simulink model "AFG_s1v1"  (R2022b)
settings: Solver=ode45  StartTime=0.0  StopTime=inf  RelTol=1e-3  EnableMultiTasking=on
values from neighbouring files (symbols this model uses):
  axle_rate_limit = 1    [call_AFG4hil_s1v1.m]
  BRAKE = [1 1 1 1 1 1 1 1]/8'    [call_AFG4hil_s1v1.m]    (also in call_AFG_s1v1.m)
  brake_lag = 0.002    [call_AFG_s1v1.m]
  brake_rate = 5000    [call_AFG_s1v1.m]
  DRIVE = [0.25 0.25  0 0 0 0 0.25 0.25]/1'    [call_AFG4hil_s1v1.m]    (also in call_AFG_s1v1.m)
  Kad = 0.0    (= 0)    [call_AFG4hil_s1v1.m]
  Kai = 0.05    [call_AFG4hil_s1v1.m]
  Kap = 0.1    [call_AFG4hil_s1v1.m]
  KDspd = 0.1    [call_AFG4hil_s1v1.m]    (also in call_AFG_s1v1.m = 0)
  KIspd = 0.1    [call_AFG4hil_s1v1.m]    (also in call_AFG_s1v1.m = 0)
  KPspd = 10    [call_AFG4hil_s1v1.m]    (also in call_AFG_s1v1.m = 20)
  Lspd = -7    [call_AFG4hil_s1v1.m]
  Nspd = 10    [call_AFG4hil_s1v1.m]
  RW = 0.499    [call_AFG4hil_s1v1.m]    (also in call_AFG_s1v1.m)
  Tb = 0.002    [call_AFG_s1v1.m]
  TRACK = temptrack    [article.m]    (also in calculate_offtrack.m; call_AFG4hil_s1v1.m = trackgen4(2,50); call_AFG_s1v1.m = trackgen4(2,50); tracktest.m)
  Tst = 0.05    [call_AFG4hil_s1v1.m]    (also in call_AFG_s1v1.m = 0.02)
  Uspd = 5    [call_AFG4hil_s1v1.m]
  vconst = 15*kph    (= 4.16666666667)    [call_AFG4hil_s1v1.m]    (also in call_AFG_s1v1.m = 5.55555555556)
undefined symbols (not defined in the file or in its folder): PARSa, PARSu, TOTALMASS
libraries: CarMaker4SL x154, slpidlib x2, TruckMaker4SL x1, simulink x1
(part 1 of 3)
settings Model: Creator=fh  LastModifiedBy=14668
settings SolverCC: AlgebraicLoopSolver=TrustRegion
settings DataIOCC: LimitDataPoints=on  SaveFormat=Array  ReturnWorkspaceOutputs=off  SignalLoggingName=sigsOut
settings OptimizationCC: BooleanDataType=off  ExpressionDepthLimit=2147483647  InitFltsAndDblsToZero=on  LifeSpan=inf
settings DebuggingCC: SaveWithParameterizedLinksMsg=none  UnderspecifiedInitializationDetection=Classic  MergeDetectMultiDrivingBlocksExec=none  SignalResolutionControl=TryResolveAllWithWarning  MultiTaskDSMMsg=warning  MultiTaskCondExecSysMsg=none  FcnCallInpInsideContextMsg=warning  UnconnectedInputMsg=warning  UnconnectedOutputMsg=warning  UnconnectedLineMsg=warning  StateNameClashWarn=warning  SFUnexpectedBacktrackingDiag=warning  SFNoUnconditionalDefaultTransitionDiag=warning  SFMachineParentedDataDiag=warning  ArithmeticOperatorsInVariantConditions=warning
settings HardwareCC: ProdBitPerPointer=32  ProdBitPerSizeT=32  ProdBitPerPtrDiffT=32  ProdLargestAtomicFloat=None  ProdIntDivRoundTo=Undefined  ProdEndianess=Unspecified  ProdWordSize=32  ProdHWDeviceType=32-bit Generic  TargetUnknown=on
settings ModelReferenceCC: EnableRefExpFcnMdlSchedulingChecks=on  PropagateSignalLabelsOutOfModel=off
settings SFSimCC: SimUseLocalCustomCode=off  CustomCodeUndefinedFunction=UseInterfaceOnly
settings RTWCC: RTWUseLocalCustomCode=off
settings CodeAppCC: MaxIdLength=63  StateflowObjectComments=on
settings GRTTargetCC: TargetFcnLib=ansi_tfl_tmw.mat  TargetLangStandard=C89/C90 (ANSI)  CombineOutputUpdateFcns=off  GRTInterface=on
settings ConfigComp: CovMetricSettings=dw  CovSaveCumulativeToWorkspaceVar=on  CovSaveSingleToWorkspaceVar=on  CovExternalEMLEnable=off

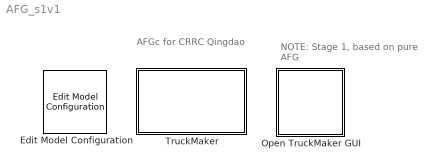
== system AFG_s1v1 ==
  note: AFGc for CRRC Qingdao
  note: NOTE:
      | Stage 1, based on pure AFG
  Edit Model Configuration : TruckMaker4SL/Edit Model Configuration  SFunctionModules=''
  Open TruckMaker GUI : Subsystem  LoadFcn=if ~length(which('cmself')), cmenv; end
      settings: OpenFcn=cmblockmagic('gui_fix_display'); TM_Simulink
      mask Display: image(imread('TruckMakerGUI.png'));
  TruckMaker : Subsystem  TreatAsAtomicUnit=on
      mask Display: image(imread('TruckMakerSys.png'));

== system AFG_s1v1/Open TruckMaker GUI ==
  S-Function : S-Function  FunctionName=cm_gui  SFunctionDeploymentMode=off  EnableBusSupport=off

== system AFG_s1v1/TruckMaker ==
  note: main code in IPG Vehicle
  CM_FIRST : Subsystem
  CM_LAST : Subsystem
  DrivMan : Subsystem
  Ground : Ground
  IPG Vehicle : Subsystem  TreatAsAtomicUnit=on
  Terminator : Terminator
  VehicleControl : Subsystem
  wires:
  VehicleControl/2(Vhcl.Model.Source) -> IPG Vehicle/2(Vhcl.Model.Source)
  VehicleControl/7(VhclCtrl.PT) -> IPG Vehicle/7(VhclCtrl.PT)
  VehicleControl/6(VhclCtrl.Brake) -> IPG Vehicle/6(VhclCtrl.Brake)
  VehicleControl/5(Vhcl.Misc) -> IPG Vehicle/5(Vhcl.Misc)
  VehicleControl/4(Vhcl.Wheel.In) -> IPG Vehicle/4(Vhcl.Wheel.In)
  VehicleControl/3(VhclCtrl.Steering) -> IPG Vehicle/3(VhclCtrl.Steering)
  VehicleControl/1(Sync_Out) -> IPG Vehicle/1(Sync_In)
  IPG Vehicle/1(Sync_Out) -> CM_LAST/1(Sync_In)
  Ground/1 -> CM_FIRST/1(Sync_In)
  CM_LAST/1(Sync_Out) -> Terminator/1
  CM_FIRST/1(Sync_Out) -> DrivMan/1(Sync_In)
  CM_FIRST/2(Env.Misc) -> DrivMan/2(Env.Misc)
  DrivMan/1(Sync_Out) -> VehicleControl/1(Sync_In)
  DrivMan/2(DrivMan.Out) -> VehicleControl/2(DrivMan.In)

== system AFG_s1v1/TruckMaker/CM_FIRST ==
  Sync_In : Inport
  BusCreator1 : BusCreator  Inputs=8
  BusCreator2 : BusCreator  Inputs=6
  Demux1 : Demux  Outputs=14
      settings: DisplayOption=none
  Environment : S-Function  FunctionName=TM_Sfun  Parameters='Environment'  SFunctionDeploymentMode=off  EnableBusSupport=off
  IoIn : S-Function  FunctionName=TM_Sfun  Parameters='IoIn'  SFunctionDeploymentMode=off  EnableBusSupport=off
  Terminator : Terminator
  Sync_Out : Outport
  Env.Misc : Outport  Port=2
  wires:
  BusCreator2/1 -> Terminator/1  "IF Environment (in)"
  BusCreator1/1 -> Env.Misc/1
  Demux1/14 -> BusCreator2/6  "Env sRoad"
  Demux1/13 -> BusCreator2/5  "Env PoI_GCS Elev"
  Demux1/12 -> BusCreator2/4  "Env PoI_GCS Lat"
  Demux1/11 -> BusCreator2/3  "Env PoI_GCS Long"
  Demux1/10 -> BusCreator2/2  "Env Time"
  Demux1/9 -> BusCreator2/1  "Env yDay"
  Demux1/8 -> BusCreator1/8  "Env WindVel_tot z"
  Demux1/7 -> BusCreator1/7  "Env WindVel_tot y"
  Demux1/6 -> BusCreator1/6  "Env WindVel_tot x"
  Demux1/5 -> BusCreator1/5  "Env SolarRadiation"
  Demux1/4 -> BusCreator1/4  "Env AirHumidity"
  Demux1/3 -> BusCreator1/3  "Env AirPressure"
  Demux1/2 -> BusCreator1/2  "Env AirDensity"
  Demux1/1 -> BusCreator1/1  "Env Temperature"
  Environment/2 -> Demux1/1
  Environment/1 -> Sync_Out/1
  IoIn/1 -> Environment/1
  Sync_In/1 -> IoIn/1

== system AFG_s1v1/TruckMaker/CM_LAST ==
  Sync_In : Inport
  CM_User : S-Function  FunctionName=TM_Sfun  Parameters='CM_User'  SFunctionDeploymentMode=off  EnableBusSupport=off
  IoOut : S-Function  FunctionName=TM_Sfun  Parameters='IoOut'  SFunctionDeploymentMode=off  EnableBusSupport=off
  Sync_Out : Outport
  wires:
  IoOut/1 -> Sync_Out/1
  CM_User/1 -> IoOut/1
  Sync_In/1 -> CM_User/1

== system AFG_s1v1/TruckMaker/DrivMan ==
  note: There's rarely a reason to override DrivMan signals.
      | Use the VehicleControl interface for this purpose.
  Sync_In : Inport
  Env.Misc : Inport  Port=2
  BusCreator : BusCreator  Inputs=17
  Demux : Demux  Outputs=17
      settings: DisplayOption=none
  DrivMan : S-Function  FunctionName=TM_Sfun  Parameters='DrivMan'  SFunctionDeploymentMode=off  EnableBusSupport=off
  Sync_Out : Outport
  DrivMan.Out : Outport  Port=2
  wires:
  Demux/17 -> BusCreator/17  "DrivMan Steering Trq"
  Demux/16 -> BusCreator/16  "DrivMan Steering AngAcc"
  Demux/15 -> BusCreator/15  "DrivMan Steering AngVel"
  Demux/14 -> BusCreator/14  "DrivMan Steering Ang"
  Demux/13 -> BusCreator/13  "DrivMan Gas"
  Demux/12 -> BusCreator/12  "DrivMan Clutch"
  Demux/11 -> BusCreator/11  "DrivMan BrakePark"
  Demux/10 -> BusCreator/10  "DrivMan Brake"
  Demux/9 -> BusCreator/9  "DrivMan GearNo"
  Demux/8 -> BusCreator/8  "DrivMan SelectorCtrl"
  Demux/7 -> BusCreator/7  "DrivMan UserSignal4"
  Demux/6 -> BusCreator/6  "DrivMan UserSignal3"
  Demux/5 -> BusCreator/5  "DrivMan UserSignal2"
  Demux/4 -> BusCreator/4  "DrivMan UserSignal1"
  Demux/3 -> BusCreator/3  "DrivMan UserSignal0"
  Demux/2 -> BusCreator/2  "DrivMan Key"
  Demux/1 -> BusCreator/1  "DrivMan SST"
  Env.Misc/1 -> DrivMan/2
  Sync_In/1 -> DrivMan/1
  DrivMan/1 -> Sync_Out/1
  BusCreator/1 -> DrivMan.Out/1
  DrivMan/2 -> Demux/1

== system AFG_s1v1/TruckMaker/IPG Vehicle ==
  Sync_In : Inport
  Vhcl.Model.Source : Inport  Port=2
  VhclCtrl.Steering : Inport  Port=3
  Vhcl.Wheel.In : Inport  Port=4
  Vhcl.Misc : Inport  Port=5
  VhclCtrl.Brake : Inport  Port=6
  VhclCtrl.PT : Inport  Port=7
  AFGc : Subsystem
  Brake : Subsystem
  CarAndTrailer : Subsystem
  DAQ for addtional VIS and DEBUG : Subsystem
  PowerTrain : Subsystem
  Stop Simulation : Stop
  VehicleSource_BuiltIn : simulink/Logic and Bit Operations/Compare To Constant  relop=~=  const=1  OutDataTypeStr=boolean  ZeroCross=off
  Sync_Out : Outport
  wires:
  VhclCtrl.PT/1 -> PowerTrain/3(VhclCtrl.PT)
  Brake/1(Sync_Out) -> PowerTrain/1(Sync_In)
  CarAndTrailer/1(Sync_Out) -> Brake/1(Sync_In)
  CarAndTrailer/2(Brake.IF.In) -> Brake/2(Brake.IF.In)
  VhclCtrl.Brake/1 -> Brake/3(VhclCtrl.Brake)
  PowerTrain/1(Sync_Out) -> Sync_Out/1
  Vhcl.Misc/1 -> CarAndTrailer/4(Vhcl.Misc)
  Vhcl.Wheel.In/1 -> CarAndTrailer/3(Vhcl.Wheel.In)
  VhclCtrl.Steering/1 -> CarAndTrailer/2(VhclCtrl.Steering)
  Sync_In/1 -> CarAndTrailer/1(Sync_In)
  Vhcl.Model.Source/1 -> VehicleSource_BuiltIn/1
  VehicleSource_BuiltIn/1 -> Stop Simulation/1
  Brake/2(Vhcl.Wheel.PT) -> PowerTrain/2(Vhcl.Wheel.PT)
  AFGc/1(tractor brake1) -> Brake/4(tractor brake)

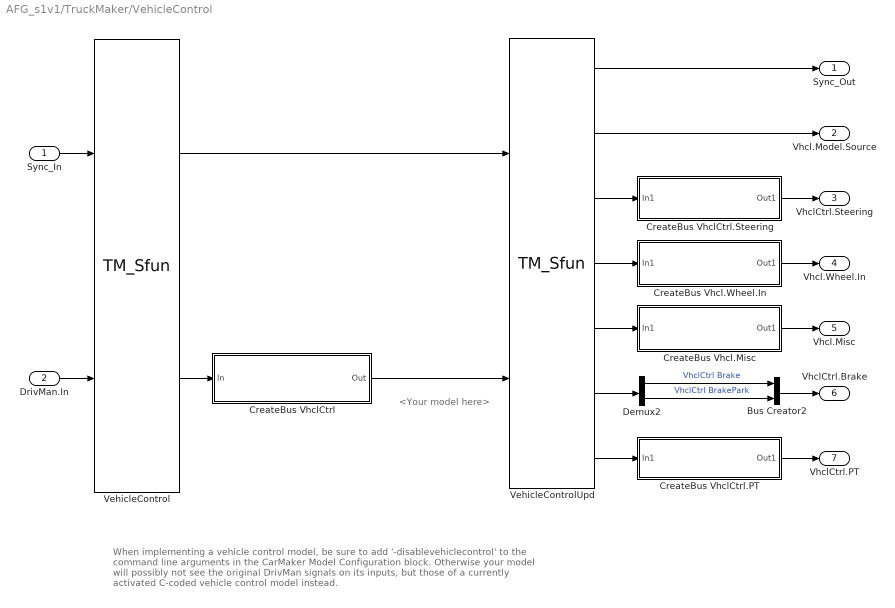
== system AFG_s1v1/TruckMaker/VehicleControl ==
  note: <Your model here>
  note: When implementing a vehicle control model,
      | be sure to add '-disablevehiclecontrol' to the command line arguments
      | in the CarMaker Model Configuration block.
      | Otherwise your model will possibly not see the original DrivMan signals
      | on its inputs, but those of a currently activated C-coded vehicle control model instead.
  Sync_In : Inport
  DrivMan.In : Inport  Port=2
  Bus Creator2 : BusCreator  Inputs=2
  CreateBus Vhcl.Misc : Subsystem
  CreateBus Vhcl.Wheel.In : Subsystem
  CreateBus VhclCtrl : Subsystem
  CreateBus VhclCtrl.PT : Subsystem
  CreateBus VhclCtrl.Steering : Subsystem
  Demux2 : Demux  Outputs=2
      settings: DisplayOption=none
  VehicleControl : S-Function  FunctionName=TM_Sfun  Parameters='VehicleControl'  SFunctionDeploymentMode=off  EnableBusSupport=off
  VehicleControlUpd : S-Function  FunctionName=TM_Sfun  Parameters='VehicleControlUpd'  SFunctionDeploymentMode=off  EnableBusSupport=off
  Sync_Out : Outport
  Vhcl.Model.Source : Outport  Port=2
  VhclCtrl.Steering : Outport  Port=3
  Vhcl.Wheel.In : Outport  Port=4
  Vhcl.Misc : Outport  Port=5
  VhclCtrl.Brake : Outport  Port=6
  VhclCtrl.PT : Outport  Port=7
  wires:
  VehicleControlUpd/2 -> Vhcl.Model.Source/1
  VehicleControlUpd/4 -> CreateBus Vhcl.Wheel.In/1(In1)
  VehicleControlUpd/5 -> CreateBus Vhcl.Misc/1(In1)
  VehicleControlUpd/6 -> Demux2/1
  VehicleControlUpd/7 -> CreateBus VhclCtrl.PT/1(In1)
  VehicleControlUpd/3 -> CreateBus VhclCtrl.Steering/1(In1)
  CreateBus Vhcl.Misc/1(Out1) -> Vhcl.Misc/1
  CreateBus Vhcl.Wheel.In/1(Out1) -> Vhcl.Wheel.In/1
  DrivMan.In/1 -> VehicleControl/2
  CreateBus VhclCtrl/1(Out) -> VehicleControlUpd/2
  VehicleControl/1 -> VehicleControlUpd/1
  VehicleControl/2 -> CreateBus VhclCtrl/1(In)
  Sync_In/1 -> VehicleControl/1
  CreateBus VhclCtrl.PT/1(Out1) -> VhclCtrl.PT/1
  Bus Creator2/1 -> VhclCtrl.Brake/1
  CreateBus VhclCtrl.Steering/1(Out1) -> VhclCtrl.Steering/1
  VehicleControlUpd/1 -> Sync_Out/1
  Demux2/2 -> Bus Creator2/2  "VhclCtrl BrakePark"
  Demux2/1 -> Bus Creator2/1  "VhclCtrl Brake"

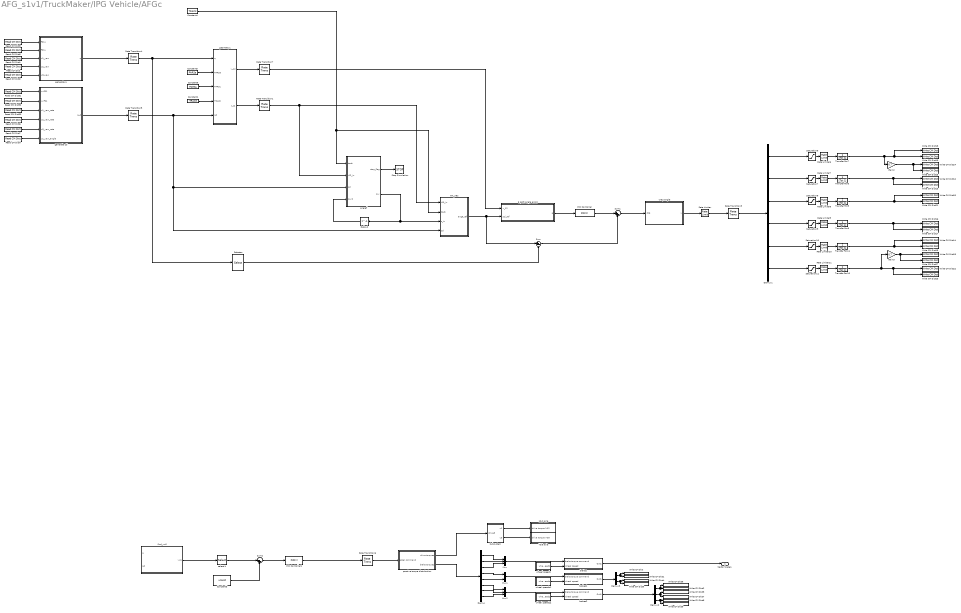
== system AFG_s1v1/TruckMaker/IPG Vehicle/AFGc ==
  1&2 axle : Subsystem
  6 path angle errors : MATLAB Function  TreatAsAtomicUnit=on
  7&8 axle : Subsystem
  Constant1 : Constant  Value=TRACK
  Constant3 : Constant  Value=vconst
  Constant4 : Constant  Value=TRACK
  Constant5 : Constant  Value=PARSa
  Constant6 : Constant  Value=PARSu
  Delay2 : Delay  DelayLength=1
  Demux : Demux  Outputs=8
  Demux1 : Demux  Outputs=6
  Demux2 : Demux  Outputs=3
  Demux3 : Demux  Outputs=2
  Gain2 : Gain  Gain=0.7
  Gain3 : Gain  Gain=0.7
  Mux : Mux  Inputs=3
  Mux1 : Mux  Inputs=2
  Mux2 : Mux  Inputs=3
  PID Controller : slpidlib/PID Controller  Controller=PID  Form=Parallel  TimeDomain=Discrete-time  UseExternalTs=off  SampleTime=-1  IntegratorMethod=Forward Euler  FilterMethod=Forward Euler  ControllerParametersSource=internal  P=Kap  I=Kai  UseKiTs=off  D=Kad  N=100  UseFilter=off  TunerSelectOption=Transfer Function Based (PID Tuner App)  InitialConditionSource=internal  InitialConditionForIntegrator=0  InitialConditionForFilter=0  DifferentiatorICPrevScaledInput=0  ExternalReset=none  TrackingMode=off  Kt=1  LimitOutput=on  SatLimitsSource=internal  UpperSaturationLimit=0.1  LowerSaturationLimit=-0.1  LinearizeAsGain=on  AntiWindupMode=clamping  Kb=1  LimitIntegrator=off  UpperIntegratorSaturationLimit=inf  LowerIntegratorSaturationLimit=-inf  POutMin=[]  POutMax=[]  IOutMin=[]  IOutMax=[]  DOutMin=[]  DOutMax=[]  NOutMin=[]  NOutMax=[]  SumOutMin=[]  SumOutMax=[]  SaturationOutMin=[]  SaturationOutMax=[]  PParamMin=[]  PParamMax=[]  IParamMin=[]  IParamMax=[]  DParamMin=[]  DParamMax=[]  NParamMin=[]  NParamMax=[]  KbParamMin=[]  KbParamMax=[]  KtParamMin=[]  KtParamMax=[]  KbOutMin=[]  KbOutMax=[]  KtOutMin=[]  KtOutMax=[]  IntegratorOutMin=[]  IntegratorOutMax=[]  FilterOutMin=[]  FilterOutMax=[]  SumI1OutMin=[]  SumI1OutMax=[]  SumI2OutMin=[]  SumI2OutMax=[]  SumI3OutMin=[]  SumI3OutMax=[]  SumI4OutMin=[]  SumI4OutMax=[]  SumDOutMin=[]  SumDOutMax=[]  DifferentiatorOutMin=[]  DifferentiatorOutMax=[]  FilterDiffOutCoefMin=[]  FilterDiffOutCoefMax=[]  ReciprocalOutMin=[]  ReciprocalOutMax=[]  SumDenOutMin=[]  SumDenOutMax=[]  SumNumOutMin=[]  SumNumOutMax=[]  DivideOutMin=[]  DivideOutMax=[]  UdiffTsProdOutMin=[]  UdiffTsProdOutMax=[]  NTsProdOutMin=[]  NTsProdOutMax=[]  UintegralTsProdOutMin=[]  UintegralTsProdOutMax=[]  UngainTsProdOutMin=[]  UngainTsProdOutMax=[]  ClampingZeroOutDataTypeStr=Inherit: Inherit via back propagation  ClampingZeroOutMin=[]  ClampingZeroOutMax=[]  FilterDenConstantOutDataTypeStr=Inherit: Inherit via back propagation  FilterDenConstantOutMin=[]  FilterDenConstantOutMax=[]  PCopyOutDataTypeStr=Inherit: Inherit via back propagation  PCopyOutMin=[]  PCopyOutMax=[]  NCopyOutDataTypeStr=Inherit: Inherit via back propagation  NCopyOutMin=[]  NCopyOutMax=[]  IntegratorContinuousStateAttributes=''  IntegratorStateMustResolveToSignalObject=off  IntegratorRTWStateStorageClass=Auto  FilterContinuousStateAttributes=''  FilterStateMustResolveToSignalObject=off  FilterRTWStateStorageClass=Auto  ParallelPVariant=InternalParameters  IdealPVariant=Disabled  IVariant=InternalParameters  DVariant=InternalParameters  IntegratorVariant=Discrete  SatVariant=Enabled  AWVariant=DiscClampingParallel  PCopyVariant=Disabled  TRVariant=Disabled  FdbkBlocksVariant=Forward  IdealPFdbkVariant=Disabled  SatFdbkVariant=Disabled  DerivativeFilterVariant=Differentiator  NVariant=Passthrough  NCopyVariant=Disabled_SignalSpec  FilterICVariant=InternalICsDifferentiator  IntegratorICVariant=InternalICs  ExternalResetVariant=Disabled  TRSumVariant=Passthrough  SumFdbkVariant=Disabled  SumVariant=Sum_PID  TsampFilterVariant=InternalTs  TsampNgainVariant=Passthrough  TsampIntegralVariant=Passthrough  ExternalSaturationOutDataTypeStr=Inherit: Same as second input
  PID Controller1 : slpidlib/PID Controller  Controller=PID  Form=Parallel  TimeDomain=Discrete-time  UseExternalTs=off  SampleTime=-1  IntegratorMethod=Forward Euler  FilterMethod=Forward Euler  ControllerParametersSource=internal  P=KPspd  I=KIspd  UseKiTs=off  D=KDspd  N=Nspd  UseFilter=on  TunerSelectOption=Transfer Function Based (PID Tuner App)  InitialConditionSource=internal  InitialConditionForIntegrator=0  InitialConditionForFilter=0  DifferentiatorICPrevScaledInput=0  ExternalReset=none  TrackingMode=off  Kt=1  LimitOutput=on  SatLimitsSource=internal  UpperSaturationLimit=Uspd  LowerSaturationLimit=Lspd  LinearizeAsGain=on  AntiWindupMode=clamping  Kb=1  LimitIntegrator=off  UpperIntegratorSaturationLimit=inf  LowerIntegratorSaturationLimit=-inf  POutMin=[]  POutMax=[]  IOutMin=[]  IOutMax=[]  DOutMin=[]  DOutMax=[]  NOutMin=[]  NOutMax=[]  SumOutMin=[]  SumOutMax=[]  SaturationOutMin=[]  SaturationOutMax=[]  PParamMin=[]  PParamMax=[]  IParamMin=[]  IParamMax=[]  DParamMin=[]  DParamMax=[]  NParamMin=[]  NParamMax=[]  KbParamMin=[]  KbParamMax=[]  KtParamMin=[]  KtParamMax=[]  KbOutMin=[]  KbOutMax=[]  KtOutMin=[]  KtOutMax=[]  IntegratorOutMin=[]  IntegratorOutMax=[]  FilterOutMin=[]  FilterOutMax=[]  SumI1OutMin=[]  SumI1OutMax=[]  SumI2OutMin=[]  SumI2OutMax=[]  SumI3OutMin=[]  SumI3OutMax=[]  SumI4OutMin=[]  SumI4OutMax=[]  SumDOutMin=[]  SumDOutMax=[]  DifferentiatorOutMin=[]  DifferentiatorOutMax=[]  FilterDiffOutCoefMin=[]  FilterDiffOutCoefMax=[]  ReciprocalOutMin=[]  ReciprocalOutMax=[]  SumDenOutMin=[]  SumDenOutMax=[]  SumNumOutMin=[]  SumNumOutMax=[]  DivideOutMin=[]  DivideOutMax=[]  UdiffTsProdOutMin=[]  UdiffTsProdOutMax=[]  NTsProdOutMin=[]  NTsProdOutMax=[]  UintegralTsProdOutMin=[]  UintegralTsProdOutMax=[]  UngainTsProdOutMin=[]  UngainTsProdOutMax=[]  ClampingZeroOutDataTypeStr=Inherit: Inherit via back propagation  ClampingZeroOutMin=[]  ClampingZeroOutMax=[]  FilterDenConstantOutDataTypeStr=Inherit: Inherit via back propagation  FilterDenConstantOutMin=[]  FilterDenConstantOutMax=[]  PCopyOutDataTypeStr=Inherit: Inherit via back propagation  PCopyOutMin=[]  PCopyOutMax=[]  NCopyOutDataTypeStr=Inherit: Inherit via back propagation  NCopyOutMin=[]  NCopyOutMax=[]  IntegratorContinuousStateAttributes=''  IntegratorStateMustResolveToSignalObject=off  IntegratorRTWStateStorageClass=Auto  FilterContinuousStateAttributes=''  FilterStateMustResolveToSignalObject=off  FilterRTWStateStorageClass=Auto  ParallelPVariant=InternalParameters  IdealPVariant=Disabled  IVariant=InternalParameters  DVariant=InternalParameters  IntegratorVariant=Discrete  SatVariant=Enabled  AWVariant=DiscClampingParallel  PCopyVariant=Disabled  TRVariant=Disabled  FdbkBlocksVariant=Forward  IdealPFdbkVariant=Disabled  SatFdbkVariant=Disabled  DerivativeFilterVariant=ForwardEulerFilter  NVariant=InternalParameters  NCopyVariant=Disabled  FilterICVariant=InternalICsFilter  IntegratorICVariant=InternalICs  ExternalResetVariant=Disabled  TRSumVariant=Passthrough  SumFdbkVariant=Disabled  SumVariant=Sum_PID  TsampFilterVariant=InternalTs  TsampNgainVariant=Passthrough  TsampIntegralVariant=Passthrough  ExternalSaturationOutDataTypeStr=Inherit: Same as second input
  Rate Limiter : RateLimiter  RisingSlewLimit=axle_rate_limit  FallingSlewLimit=-axle_rate_limit  SampleTimeMode=inherited
  Rate Limiter{6..11} (6 alike) : RateLimiter  RisingSlewLimit=3  FallingSlewLimit=-3  SampleTimeMode=inherited
  Rate Transition{1,3..7} (6 alike) : RateTransition
  Read CM Dict : CarMaker4SL/Read CM Dict  xname=Tr.Yaw  xsync=off  xstime=Continuous
  Read CM Dict1 : CarMaker4SL/Read CM Dict  xname=Car.Yaw  xsync=off  xstime=Continuous
  Read CM Dict2 : CarMaker4SL/Read CM Dict  xname=Tr2.Yaw  xsync=off  xstime=Continuous
  Read CM Dict3 : CarMaker4SL/Read CM Dict  xname=Car.Fr1.tx  xsync=off  xstime=Continuous
  Read CM Dict30 : CarMaker4SL/Read CM Dict  xname=Car.YawRate  xsync=off  xstime=Continuous
  Read CM Dict31 : CarMaker4SL/Read CM Dict  xname=Car.Fr1.vx  xsync=off  xstime=Continuous
  Read CM Dict32 : CarMaker4SL/Read CM Dict  xname=Car.Fr1.vy  xsync=off  xstime=Continuous
  Read CM Dict4 : CarMaker4SL/Read CM Dict  xname=Car.Yaw  xsync=off  xstime=Continuous
  Read CM Dict5 : CarMaker4SL/Read CM Dict  xname=Car.Fr1.ty  xsync=off  xstime=Continuous
  Read CM Dict6 : CarMaker4SL/Read CM Dict  xname=Tr.YawVel  xsync=off  xstime=Continuous
  Read CM Dict7 : CarMaker4SL/Read CM Dict  xname=Tr2.YawVel  xsync=off  xstime=Continuous
  Saturation10 : Saturate  UpperLimit=0.3491  LowerLimit=-0.3491
  Saturation11 : Saturate  UpperLimit=0.2443  LowerLimit=-0.2443
  Saturation6 : Saturate  UpperLimit=0.3491  LowerLimit=-0.3491
  Saturation7 : Saturate  UpperLimit=0.2443  LowerLimit=-0.2443
  Saturation8 : Saturate  UpperLimit=0.3491  LowerLimit=-0.3491
  Saturation9 : Saturate  UpperLimit=0.2443  LowerLimit=-0.2443
  Selector : Selector  InputPortWidth=5  IndexOptions=Index vector (dialog)  Indices=[3 3 4 4 5 5]  OutputSizes=1
  Stop Simulation : Stop
  Subsystem : Subsystem
  Sum : Sum  Inputs=|+-
  Sum1 : Sum  Inputs=|++
  Sum2 : Sum  Inputs=|-+
  Transfer Fcn{6..11} (6 alike) : TransferFcn  Denominator=[Tst 1]
  WK_w8s : MATLAB Function  TreatAsAtomicUnit=on
  Write CM Dict : CarMaker4SL/Write CM Dict  xname=Tr.Brake.Trq_FL_ext  xsync=off
  Write CM Dict1 : CarMaker4SL/Write CM Dict  xname=Tr.Brake.Trq_FR_ext  xsync=off
  Write CM Dict12 : CarMaker4SL/Write CM Dict  xname=Car.CRL2.rz_ext  xsync=off
  Write CM Dict13 : CarMaker4SL/Write CM Dict  xname=Car.CRR2.rz_ext  xsync=off
  Write CM Dict14 : CarMaker4SL/Write CM Dict  xname=Tr2.CFL.rz_ext  xsync=off
  Write CM Dict15 : CarMaker4SL/Write CM Dict  xname=Tr2.CFR.rz_ext  xsync=off
  Write CM Dict16 : CarMaker4SL/Write CM Dict  xname=Tr.CRL.rz_ext  xsync=off
  Write CM Dict17 : CarMaker4SL/Write CM Dict  xname=Tr.CRR.rz_ext  xsync=off
  Write CM Dict18 : CarMaker4SL/Write CM Dict  xname=Car.CFL.rz_ext  xsync=off
  Write CM Dict19 : CarMaker4SL/Write CM Dict  xname=Car.CFR.rz_ext  xsync=off
  Write CM Dict2 : CarMaker4SL/Write CM Dict  xname=Tr2.Brake.Trq_FR_ext  xsync=off
  Write CM Dict20 : CarMaker4SL/Write CM Dict  xname=Tr.CFL.rz_ext  xsync=off
  Write CM Dict21 : CarMaker4SL/Write CM Dict  xname=Tr.CFR.rz_ext  xsync=off
  Write CM Dict22 : CarMaker4SL/Write CM Dict  xname=Tr2.CRL.rz_ext  xsync=off
  Write CM Dict23 : CarMaker4SL/Write CM Dict  xname=Tr2.CRR.rz_ext  xsync=off
  Write CM Dict24 : CarMaker4SL/Write CM Dict  xname=Car.CRL.rz_ext  xsync=off
  Write CM Dict25 : CarMaker4SL/Write CM Dict  xname=Car.CRR.rz_ext  xsync=off
  Write CM Dict26 : CarMaker4SL/Write CM Dict  xname=Tr2.CML.rz_ext  xsync=off
  Write CM Dict27 : CarMaker4SL/Write CM Dict  xname=Tr2.CMR.rz_ext  xsync=off
  Write CM Dict3 : CarMaker4SL/Write CM Dict  xname=Tr2.Brake.Trq_ML_ext  xsync=off
  Write CM Dict4 : CarMaker4SL/Write CM Dict  xname=Tr.Brake.Trq_RL_ext  xsync=off
  Write CM Dict5 : CarMaker4SL/Write CM Dict  xname=Tr.Brake.Trq_RR_ext  xsync=off
  Write CM Dict6 : CarMaker4SL/Write CM Dict  xname=Tr2.Brake.Trq_FL_ext  xsync=off
  Write CM Dict7 : CarMaker4SL/Write CM Dict  xname=Tr2.Brake.Trq_MR_ext  xsync=off
  Write CM Dict8 : CarMaker4SL/Write CM Dict  xname=Tr2.Brake.Trq_RL_ext  xsync=off
  Write CM Dict9 : CarMaker4SL/Write CM Dict  xname=Tr2.Brake.Trq_RR_ext  xsync=off
  angref : MATLAB Function  TreatAsAtomicUnit=on
  brakes : Subsystem
  brakes1 : Subsystem
  brakes2 : Subsystem
  find_vx6 : MATLAB Function  TreatAsAtomicUnit=on
  generate q : MATLAB Function  TreatAsAtomicUnit=on
  generate qd : MATLAB Function  TreatAsAtomicUnit=on
  geometry1 : MATLAB Function  TreatAsAtomicUnit=on
  passive torque distrubution : Subsystem
  select U : Selector  InputPortWidth=6  IndexOptions=Index vector (dialog)  Indices=[1]  OutputSizes=1
  wheel speeds : Subsystem
  wheel speeds1 : Subsystem
  wheel speeds2 : Subsystem
  wrap angle : MATLAB Function  TreatAsAtomicUnit=on
  tractor brake1 : Outport  VectorParamsAs1DForOutWhenUnconnected=off
  wires:
  Read CM Dict5/1 -> generate q/2(FR1y)
  Read CM Dict2/1 -> generate q/5(u3_yaw)
  Read CM Dict1/1 -> generate q/3(u1_yaw)
  Read CM Dict/1 -> generate q/4(u2_yaw)
  Read CM Dict3/1 -> generate q/1(FR1x)
  Read CM Dict6/1 -> generate qd/4(u2_yaw_rate)
  Read CM Dict30/1 -> generate qd/3(u1_yaw_rate)
  Read CM Dict32/1 -> generate qd/2(vyFR1)
  Read CM Dict7/1 -> generate qd/5(u3_yaw_rate)
  Read CM Dict31/1 -> generate qd/1(vxFR1)
  Read CM Dict4/1 -> generate qd/6(u1_yaw_angle)
  Demux1/6 -> Saturation11/1
  Rate Limiter10/1 -> Transfer Fcn11/1
  Rate Limiter8/1 -> Transfer Fcn9/1
  Saturation10/1 -> Rate Limiter10/1
  Saturation11/1 -> Rate Limiter11/1
  Saturation9/1 -> Rate Limiter9/1
  Gain2/1 -> Write CM Dict25/1, Write CM Dict24/1
  Demux1/5 -> Saturation10/1
  Rate Transition3/1 -> Demux1/1
  Saturation8/1 -> Rate Limiter8/1
  Transfer Fcn6/1 -> Write CM Dict13/1, Write CM Dict12/1
  Transfer Fcn7/1 -> Write CM Dict18/1, Write CM Dict19/1, Gain2/1
  Transfer Fcn9/1 -> Write CM Dict20/1, Write CM Dict21/1
  Saturation7/1 -> Rate Limiter7/1
  Rate Limiter6/1 -> Transfer Fcn7/1
  Saturation6/1 -> Rate Limiter6/1
  Demux1/3 -> Saturation8/1
  Gain3/1 -> Write CM Dict27/1, Write CM Dict26/1
  Demux1/1 -> Saturation6/1
  Transfer Fcn11/1 -> Write CM Dict14/1, Write CM Dict15/1
  Rate Limiter11/1 -> Transfer Fcn10/1
  Transfer Fcn10/1 -> Write CM Dict23/1, Write CM Dict22/1, Gain3/1
  Rate Limiter7/1 -> Transfer Fcn6/1
  Demux1/2 -> Saturation7/1
  Demux1/4 -> Saturation9/1
  Rate Limiter9/1 -> Transfer Fcn8/1
  Transfer Fcn8/1 -> Write CM Dict17/1, Write CM Dict16/1
  Demux/7 -> Mux2/2
  passive torque distrubution/1(drive torques) -> Subsystem/1(drive8)
  Demux2/3 -> Write CM Dict9/1, Write CM Dict8/1
  Demux/8 -> Mux2/3
  brakes2/1(Out1) -> Demux2/1
  Demux3/1 -> Write CM Dict/1, Write CM Dict1/1
  Demux/2 -> Mux/2
  Subsystem/2(u3) -> 7&8 axle/1(drive torque 7&8)
  Mux2/1 -> brakes2/1(brake torque command)
  brakes1/1(Out1) -> Demux3/1
  Demux2/1 -> Write CM Dict2/1, Write CM Dict6/1
  Mux/1 -> brakes/1(brake torque command)
  Mux1/1 -> brakes1/1(brake torque command)
  Demux/6 -> Mux2/1
  Demux/4 -> Mux1/1
  Demux/3 -> Mux/3
  wheel speeds2/1(wheel speeds) -> brakes2/2(wheel speed)
  Demux/5 -> Mux1/2
  brakes/1(Out1) -> tractor brake1/1
  Demux2/2 -> Write CM Dict7/1, Write CM Dict3/1
  Demux3/2 -> Write CM Dict4/1, Write CM Dict5/1
  wheel speeds/1(wheel speeds) -> brakes/2(wheel speed)
  wheel speeds1/1(wheel speeds) -> brakes1/2(wheel speed)
  Demux/1 -> Mux/1
  passive torque distrubution/2(brake torques) -> Demux/1
  Subsystem/1(u1) -> 1&2 axle/1(drive torque 1&2)
  Constant1/1 -> geometry1/4(TRACK)
  Constant5/1 -> geometry1/2(PARSa)
  geometry1/2(r_12) -> Rate Transition1/1
  geometry1/1(v_12) -> Rate Transition7/1
  Constant6/1 -> geometry1/3(PARSu)
  Rate Transition7/1 -> 6 path angle errors/1(v_12)
  Sum1/1 -> wrap angle/1(str6)
  Rate Transition4/1 -> Selector/1, geometry1/1(q)
  Selector/1 -> Sum/2
  wrap angle/1(y) -> Rate Limiter/1
  Rate Transition5/1 -> WK_w8s/4(qd), angref/3(qd), geometry1/5(qd)
  WK_w8s/1(ang6_ref) -> Sum/1, 6 path angle errors/2(psi_ref)
  generate q/1(q) -> Rate Transition4/1
  generate qd/1(q_d) -> Rate Transition5/1
  Delay2/1 -> angref/4(sxy0)
  angref/2(sxy) -> Delay2/1, WK_w8s/3(s_in)
  Constant4/1 -> angref/1(track), WK_w8s/2(track)
  angref/1(stop_flag) -> Stop Simulation/1
  select U/1 -> Sum2/1
  Sum2/1 -> PID Controller1/1
  find_vx6/1(vx6) -> select U/1
  Constant3/1 -> Sum2/2
  PID Controller1/1 -> Rate Transition6/1
  6 path angle errors/1(e) -> PID Controller/1
  PID Controller/1 -> Sum1/1
  Sum/1 -> Sum1/2
  Rate Transition6/1 -> passive torque distrubution/1(accel command)
  Rate Limiter/1 -> Rate Transition3/1
  Rate Transition1/1 -> angref/2(r12_in), WK_w8s/1(r10_in)

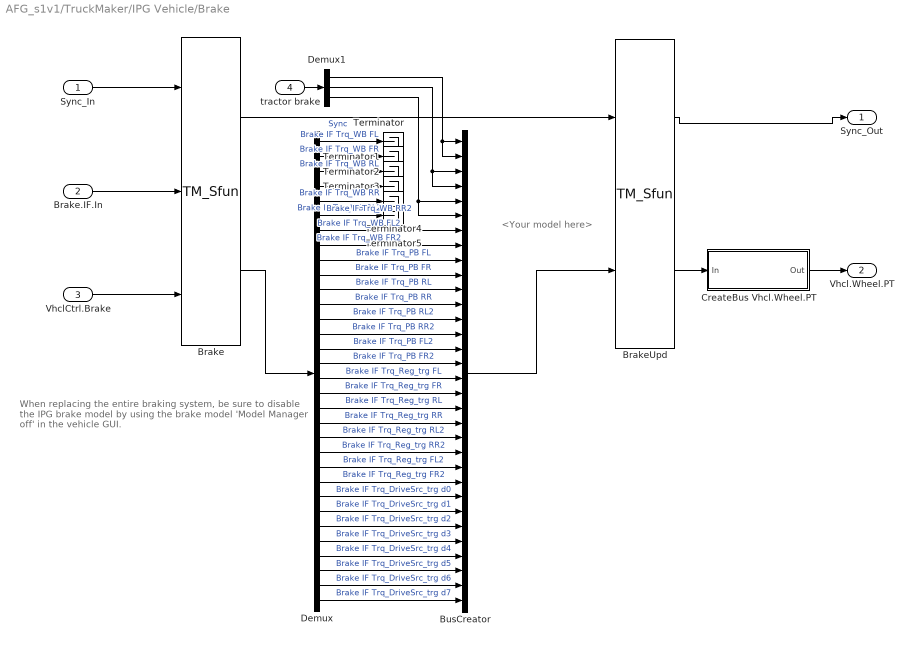
== system AFG_s1v1/TruckMaker/IPG Vehicle/Brake ==
  note: <Your model here>
  note: When replacing the entire braking system,
      | be sure to disable the IPG brake model by using the brake
      | model 'Model Manager off' in the vehicle GUI.
  Sync_In : Inport
  Brake.IF.In : Inport  Port=2
  VhclCtrl.Brake : Inport  Port=3
  tractor brake : Inport  Port=4
  Brake : S-Function  FunctionName=TM_Sfun  Parameters='Brake'  SFunctionDeploymentMode=off  EnableBusSupport=off
  BrakeUpd : S-Function  FunctionName=TM_Sfun  Parameters='BrakeUpd'  SFunctionDeploymentMode=off  EnableBusSupport=off
  BusCreator : BusCreator  Inputs=32
  CreateBus Vhcl.Wheel.PT : Subsystem
  Demux : Demux  Outputs=32
      settings: DisplayOption=none
  Demux1 : Demux  Outputs=3
  Terminator{,1..5} (6 alike) : Terminator
  Sync_Out : Outport
  Vhcl.Wheel.PT : Outport  Port=2
  wires:
  Demux/32 -> BusCreator/32  "Brake IF Trq_DriveSrc_trg d7"
  Demux/31 -> BusCreator/31  "Brake IF Trq_DriveSrc_trg d6"
  Demux/30 -> BusCreator/30  "Brake IF Trq_DriveSrc_trg d5"
  Demux/29 -> BusCreator/29  "Brake IF Trq_DriveSrc_trg d4"
  Demux/28 -> BusCreator/28  "Brake IF Trq_DriveSrc_trg d3"
  Demux/27 -> BusCreator/27  "Brake IF Trq_DriveSrc_trg d2"
  Demux/26 -> BusCreator/26  "Brake IF Trq_DriveSrc_trg d1"
  Demux/25 -> BusCreator/25  "Brake IF Trq_DriveSrc_trg d0"
  Demux/24 -> BusCreator/24  "Brake IF Trq_Reg_trg FR2"
  Demux/23 -> BusCreator/23  "Brake IF Trq_Reg_trg FL2"
  Demux/22 -> BusCreator/22  "Brake IF Trq_Reg_trg RR2"
  Demux/21 -> BusCreator/21  "Brake IF Trq_Reg_trg RL2"
  Demux/20 -> BusCreator/20  "Brake IF Trq_Reg_trg RR"
  Demux/19 -> BusCreator/19  "Brake IF Trq_Reg_trg RL"
  Demux/18 -> BusCreator/18  "Brake IF Trq_Reg_trg FR"
  Demux/17 -> BusCreator/17  "Brake IF Trq_Reg_trg FL"
  Demux/16 -> BusCreator/16  "Brake IF Trq_PB FR2"
  Demux/15 -> BusCreator/15  "Brake IF Trq_PB FL2"
  Demux/14 -> BusCreator/14  "Brake IF Trq_PB RR2"
  Demux/13 -> BusCreator/13  "Brake IF Trq_PB RL2"
  Demux/12 -> BusCreator/12  "Brake IF Trq_PB RR"
  Demux/11 -> BusCreator/11  "Brake IF Trq_PB RL"
  Demux/10 -> BusCreator/10  "Brake IF Trq_PB FR"
  Demux/9 -> BusCreator/9  "Brake IF Trq_PB FL"
  Demux/8 -> BusCreator/8  "Brake IF Trq_WB FR2"
  Demux/7 -> BusCreator/7  "Brake IF Trq_WB FL2"
  BusCreator/1 -> BrakeUpd/2
  Brake/2 -> Demux/1
  BrakeUpd/1 -> Sync_Out/1
  Brake/1 -> BrakeUpd/1  "Sync"
  Brake.IF.In/1 -> Brake/2
  VhclCtrl.Brake/1 -> Brake/3
  Sync_In/1 -> Brake/1
  BrakeUpd/2 -> CreateBus Vhcl.Wheel.PT/1(In)
  CreateBus Vhcl.Wheel.PT/1(Out) -> Vhcl.Wheel.PT/1
  Demux1/2 -> BusCreator/3, BusCreator/4
  Demux1/1 -> BusCreator/1, BusCreator/2
  tractor brake/1 -> Demux1/1
  Demux/4 -> Terminator3/1  "Brake IF Trq_WB RR"
  Demux/3 -> Terminator2/1  "Brake IF Trq_WB RL"
  Demux/2 -> Terminator1/1  "Brake IF Trq_WB FR"
  Demux/1 -> Terminator/1  "Brake IF Trq_WB FL"
  Demux/5 -> Terminator4/1  "Brake IF Trq_WB RL2"
  Demux/6 -> Terminator5/1  "Brake IF Trq_WB RR2"
  Demux1/3 -> BusCreator/5, BusCreator/6

== system AFG_s1v1/TruckMaker/IPG Vehicle/CarAndTrailer ==
  Sync_In : Inport
  VhclCtrl.Steering : Inport  Port=2
  Vhcl.Wheel.In : Inport  Port=3
  Vhcl.Misc : Inport  Port=4
  CarAndTrailerUpd : Subsystem
  Forces : Subsystem
  Ground : Ground
  Kinematics : Subsystem
  Kinetics : Subsystem
  Steering : Subsystem
  Terminator : Terminator
  Terminator1 : Terminator
  Trailer : Subsystem
  Sync_Out : Outport
  Brake.IF.In : Outport  Port=2
  wires:
  Ground/1 -> CarAndTrailerUpd/14(Vhcl.Fr1A)
  Trailer/13(Car.Hitch.FrcTrq) -> CarAndTrailerUpd/13(Car.Hitch.FrcTrq)
  Trailer/12(Vhcl.Wheel.FR2) -> CarAndTrailerUpd/12(Vhcl.Wheel.FR2)
  Trailer/11(Vhcl.Wheel.FL2) -> CarAndTrailerUpd/11(Vhcl.Wheel.FL2)
  Trailer/10(Vhcl.Wheel.RR2) -> CarAndTrailerUpd/10(Vhcl.Wheel.RR2)
  Trailer/9(Vhcl.Wheel.RL2) -> CarAndTrailerUpd/9(Vhcl.Wheel.RL2)
  Trailer/8(Vhcl.Wheel.RR) -> CarAndTrailerUpd/8(Vhcl.Wheel.RR)
  Trailer/7(Vhcl.Wheel.RL) -> CarAndTrailerUpd/7(Vhcl.Wheel.RL)
  Trailer/6(Vhcl.Wheel.FR) -> CarAndTrailerUpd/6(Vhcl.Wheel.FR)
  Trailer/5(Vhcl.Wheel.FL) -> CarAndTrailerUpd/5(Vhcl.Wheel.FL)
  Trailer/4(Vhcl.PoI) -> CarAndTrailerUpd/4(Vhcl.PoI)
  Trailer/3(Vhcl.Motion) -> CarAndTrailerUpd/3(Vhcl.Motion)
  Trailer/2(Vhcl.Steering) -> CarAndTrailerUpd/2(Vhcl.Steering)
  Trailer/1(Sync_Out) -> CarAndTrailerUpd/1(Sync_In)
  CarAndTrailerUpd/2(Brake.IF.In) -> Brake.IF.In/1
  CarAndTrailerUpd/1(Sync_Out) -> Sync_Out/1
  Vhcl.Misc/1 -> Terminator1/1
  Vhcl.Wheel.In/1 -> Terminator/1
  Kinetics/6(WheelCarrier.Misc) -> Trailer/6(WheelCarrier.Misc)
  Kinetics/5(Car.Trq_T2W) -> Trailer/5(Car.Trq_T2W)
  Steering/2(Steer.IF) -> Kinematics/2(Steer.IF)
  Kinetics/4(Car.Fr1) -> Trailer/4(Car.Fr1)
  Kinetics/3(Car.Hitch) -> Trailer/3(Car.Hitch)
  Kinetics/2(Trailer.Load) -> Trailer/2(Trailer.Load)
  VhclCtrl.Steering/1 -> Steering/2(VhclCtrl.Steering)
  Sync_In/1 -> Steering/1(Sync_In)
  Steering/1(Sync_Out) -> Kinematics/1(Sync_In)
  Kinetics/1(Sync_Out) -> Trailer/1(Sync_In)
  Kinematics/5(lBuf) -> Forces/5(lBuf)
  Forces/8(FBuf_ext) -> Kinetics/8(FBuf_ext)
  Forces/4(Car.Load) -> Kinetics/4(Car.Load)
  Forces/7(FStabi_ext) -> Kinetics/7(FStabi_ext)
  Forces/6(FDamp_ext) -> Kinetics/6(FDamp_ext)
  Forces/5(FSpring_ext) -> Kinetics/5(FSpring_ext)
  Forces/2(Car.Virtual) -> Kinetics/2(Car.Virtual)
  Kinematics/2(lSpring) -> Forces/2(lSpring)
  Kinematics/3(vDamp) -> Forces/3(vDamp)
  Forces/3(Car.Aero) -> Kinetics/3(Car.Aero)
  Forces/1(Sync_Out) -> Kinetics/1(Sync_In)
  Kinematics/1(Sync_Out) -> Forces/1(Sync_In)
  Kinematics/4(lStabi) -> Forces/4(lStabi)

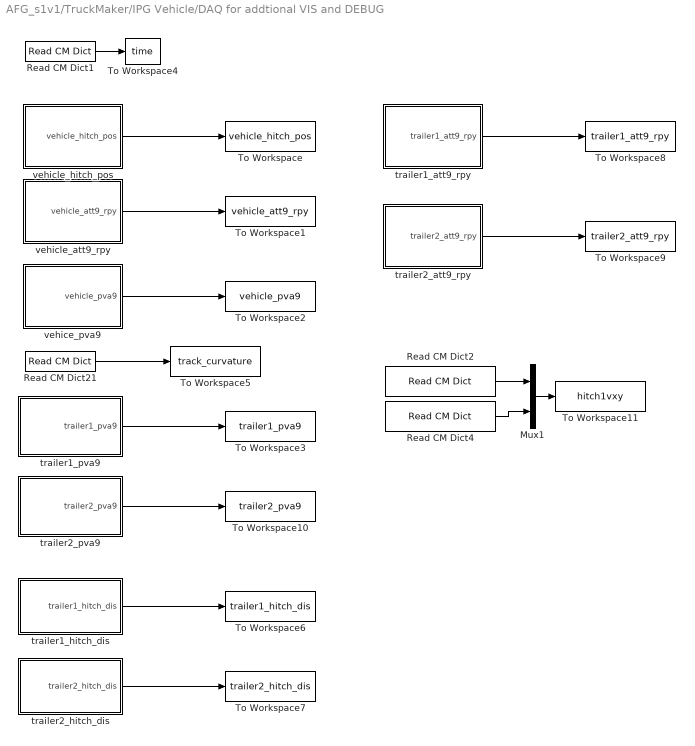
== system AFG_s1v1/TruckMaker/IPG Vehicle/DAQ for addtional VIS and DEBUG ==
  Mux1 : Mux  Inputs=2
  Read CM Dict1 : CarMaker4SL/Read CM Dict  xname=Time  xsync=off  xstime=Continuous
  Read CM Dict2 : CarMaker4SL/Read CM Dict  xname=Car.Hitch.vx  xsync=off  xstime=Continuous
  Read CM Dict21 : CarMaker4SL/Read CM Dict  xname=Car.TrackCurv  xsync=off  xstime=Continuous
  Read CM Dict4 : CarMaker4SL/Read CM Dict  xname=Car.Hitch.vy  xsync=off  xstime=Continuous
  To Workspace : ToWorkspace  VariableName=vehicle_hitch_pos  SampleTime=-1
  To Workspace1 : ToWorkspace  VariableName=vehicle_att9_rpy  SampleTime=-1
  To Workspace10 : ToWorkspace  VariableName=trailer2_pva9  SampleTime=-1
  To Workspace11 : ToWorkspace  VariableName=hitch1vxy  SampleTime=-1
  To Workspace2 : ToWorkspace  VariableName=vehicle_pva9  SampleTime=-1
  To Workspace3 : ToWorkspace  VariableName=trailer1_pva9  SampleTime=-1
  To Workspace4 : ToWorkspace  VariableName=time  SampleTime=-1
  To Workspace5 : ToWorkspace  VariableName=track_curvature  SampleTime=-1
  To Workspace6 : ToWorkspace  VariableName=trailer1_hitch_dis  SampleTime=-1
  To Workspace7 : ToWorkspace  VariableName=trailer2_hitch_dis  SampleTime=-1
  To Workspace8 : ToWorkspace  VariableName=trailer1_att9_rpy  SampleTime=-1
  To Workspace9 : ToWorkspace  VariableName=trailer2_att9_rpy  SampleTime=-1
  trailer1_att9_rpy : Subsystem
  trailer1_hitch_dis : Subsystem
  trailer1_pva9 : Subsystem
  trailer2_att9_rpy : Subsystem
  trailer2_hitch_dis : Subsystem
  trailer2_pva9 : Subsystem
  vehice_pva9 : Subsystem
  vehicle_att9_rpy : Subsystem
  vehicle_hitch_pos : Subsystem
  wires:
  vehicle_hitch_pos/1(vehicle_hitch_pos) -> To Workspace/1
  vehicle_att9_rpy/1(vehicle_att9_rpy) -> To Workspace1/1
  vehice_pva9/1(vehicle_pva9) -> To Workspace2/1
  trailer1_pva9/1(trailer1_pva9) -> To Workspace3/1
  Read CM Dict1/1 -> To Workspace4/1
  Read CM Dict21/1 -> To Workspace5/1
  trailer1_hitch_dis/1(trailer1_hitch_dis) -> To Workspace6/1
  trailer2_hitch_dis/1(trailer2_hitch_dis) -> To Workspace7/1
  trailer1_att9_rpy/1(trailer1_att9_rpy) -> To Workspace8/1
  trailer2_att9_rpy/1(trailer2_att9_rpy) -> To Workspace9/1
  trailer2_pva9/1(trailer2_pva9) -> To Workspace10/1
  Read CM Dict2/1 -> Mux1/1
  Read CM Dict4/1 -> Mux1/2
  Mux1/1 -> To Workspace11/1

== system AFG_s1v1/TruckMaker/IPG Vehicle/PowerTrain ==
  note: When replacing the entire powertrain,
      | be sure to disable the IPG powertrain model by using the powertrain
      | model 'Model Manager off' in the vehicle GUI.
  note: <Your model here>
  Sync_In : Inport
  Vhcl.Wheel.PT : Inport  Port=2
  VhclCtrl.PT : Inport  Port=3
  BusCreator : BusCreator  Inputs=70
  Demux : Demux  Outputs=70
      settings: DisplayOption=none
  PowerTrain : S-Function  FunctionName=TM_Sfun  Parameters='PowerTrain'  SFunctionDeploymentMode=off  EnableBusSupport=off
  PowerTrainUpd : S-Function  FunctionName=TM_Sfun  Parameters='PowerTrainUpd'  SFunctionDeploymentMode=off  EnableBusSupport=off
  Sync_Out : Outport
  wires:
  Demux/70 -> BusCreator/70  "PT IF WFR2 Trq_BrakeReg_max"
  Demux/69 -> BusCreator/69  "PT IF WFR2 Trq_BrakeReg"
  Demux/68 -> BusCreator/68  "PT IF WFR2 Trq_Supp2WC"
  Demux/67 -> BusCreator/67  "PT IF WFR2 Trq_Drive"
  Demux/66 -> BusCreator/66  "PT IF WFR2 Trq_B2W"
  Demux/65 -> BusCreator/65  "PT IF WFR2 rotv"
  Demux/64 -> BusCreator/64  "PT IF WFR2 rot"
  Demux/63 -> BusCreator/63  "PT IF WFL2 Trq_BrakeReg_max"
  Demux/62 -> BusCreator/62  "PT IF WFL2 Trq_BrakeReg"
  Demux/59 -> BusCreator/59  "PT IF WFL2 Trq_B2W"
  Demux/58 -> BusCreator/58  "PT IF WFL2 rotv"
  Demux/57 -> BusCreator/57  "PT IF WFL2 rot"
  Demux/56 -> BusCreator/56  "PT IF WRR2 Trq_BrakeReg_max"
  Demux/55 -> BusCreator/55  "PT IF WRR2 Trq_BrakeReg"
  Demux/52 -> BusCreator/52  "PT IF WRR2 Trq_B2W"
  Demux/51 -> BusCreator/51  "PT IF WRR2 rotv"
  Demux/50 -> BusCreator/50  "PT IF WRR2 rot"
  Demux/49 -> BusCreator/49  "PT IF WRL2 Trq_BrakeReg_max"
  Demux/48 -> BusCreator/48  "PT IF WRL2 Trq_BrakeReg"
  Demux/45 -> BusCreator/45  "PT IF WRL2 Trq_B2W"
  Demux/44 -> BusCreator/44  "PT IF WRL2 rotv"
  Demux/43 -> BusCreator/43  "PT IF WRL2 rot"
  Demux/42 -> BusCreator/42  "PT IF WRR Trq_BrakeReg_max"
  Demux/41 -> BusCreator/41  "PT IF WRR Trq_BrakeReg"
  Demux/38 -> BusCreator/38  "PT IF WRR Trq_B2W"
  Demux/37 -> BusCreator/37  "PT IF WRR rotv"
  Demux/36 -> BusCreator/36  "PT IF WRR rot"
  Demux/35 -> BusCreator/35  "PT IF WRL Trq_BrakeReg_max"
  Demux/34 -> BusCreator/34  "PT IF WRL Trq_BrakeReg"
  Demux/31 -> BusCreator/31  "PT IF WRL Trq_B2W"
  Demux/30 -> BusCreator/30  "PT IF WRL rotv"
  Demux/29 -> BusCreator/29  "PT IF WRL rot"
  Demux/28 -> BusCreator/28  "PT IF WFR Trq_BrakeReg_max"
  Demux/27 -> BusCreator/27  "PT IF WFR Trq_BrakeReg"
  Demux/24 -> BusCreator/24  "PT IF WFR Trq_B2W"
  Demux/23 -> BusCreator/23  "PT IF WFR rotv"
  Demux/22 -> BusCreator/22  "PT IF WFR rot"
  Demux/21 -> BusCreator/21  "PT IF WFL Trq_BrakeReg_max"
  Demux/20 -> BusCreator/20  "PT IF WFL Trq_BrakeReg"
  Demux/17 -> BusCreator/17  "PT IF WFL Trq_B2W"
  Demux/16 -> BusCreator/16  "PT IF WFL rotv"
  Demux/15 -> BusCreator/15  "PT IF WFL rot"
  Demux/14 -> BusCreator/14  "PT IF DL_iDiff_mean"
  Demux/13 -> BusCreator/13  "PT IF Trq_Supp2BdyEng y"
  Demux/12 -> BusCreator/12  "PT IF Trq_Supp2BdyEng x"
  Demux/11 -> BusCreator/11  "PT IF Trq_Supp2Bdy1B z"
  Demux/10 -> BusCreator/10  "PT IF Trq_Supp2Bdy1B y"
  Demux/9 -> BusCreator/9  "PT IF Trq_Supp2Bdy1B x"
  Demux/8 -> BusCreator/8  "PT IF Trq_Supp2Bdy1 z"
  Demux/7 -> BusCreator/7  "PT IF Trq_Supp2Bdy1 y"
  Demux/6 -> BusCreator/6  "PT IF Trq_Supp2Bdy1 x"
  Demux/5 -> BusCreator/5  "PT IF Engine_rotv"
  Demux/4 -> BusCreator/4  "PT IF GearNo"
  Demux/3 -> BusCreator/3  "PT IF OperationError"
  Demux/2 -> BusCreator/2  "PT IF OperationState"
  Demux/1 -> BusCreator/1  "PT IF Ignition"
  BusCreator/1 -> PowerTrainUpd/2
  PowerTrain/2 -> Demux/1
  Sync_In/1 -> PowerTrain/1
  PowerTrainUpd/1 -> Sync_Out/1
  PowerTrain/1 -> PowerTrainUpd/1  "Sync"
  VhclCtrl.PT/1 -> PowerTrain/3
  Vhcl.Wheel.PT/1 -> PowerTrain/2
  Demux/60 -> BusCreator/60  "PT IF WFL2 Trq_Drive"
  Demux/61 -> BusCreator/61  "PT IF WFL2 Trq_Supp2WC"
  Demux/18 -> BusCreator/18  "PT IF WFL Trq_Drive"
  Demux/19 -> BusCreator/19  "PT IF WFL Trq_Supp2WC"
  Demux/25 -> BusCreator/25  "PT IF WFR Trq_Drive"
  Demux/26 -> BusCreator/26  "PT IF WFR Trq_Supp2WC"
  Demux/32 -> BusCreator/32  "PT IF WRL Trq_Drive"
  Demux/33 -> BusCreator/33  "PT IF WRL Trq_Supp2WC"
  Demux/39 -> BusCreator/39  "PT IF WRR Trq_Drive"
  Demux/40 -> BusCreator/40  "PT IF WRR Trq_Supp2WC"
  Demux/46 -> BusCreator/46  "PT IF WRL2 Trq_Drive"
  Demux/47 -> BusCreator/47  "PT IF WRL2 Trq_Supp2WC"
  Demux/53 -> BusCreator/53  "PT IF WRR2 Trq_Drive"
  Demux/54 -> BusCreator/54  "PT IF WRR2 Trq_Supp2WC"

== system AFG_s1v1/TruckMaker/VehicleControl/CreateBus Vhcl.Misc ==
  In1 : Inport
  Bus Creator5 : BusCreator  Inputs=11
  Demux5 : Demux  Outputs=11
      settings: DisplayOption=none
  Out1 : Outport
  wires:
  Demux5/11 -> Bus Creator5/11  "Vhcl Wind_vel_0 z"
  Demux5/10 -> Bus Creator5/10  "Vhcl Wind_vel_0 y"
  Demux5/9 -> Bus Creator5/9  "Vhcl Wind_vel_0 x"
  Demux5/8 -> Bus Creator5/8  "Vhcl DL2BdyEng y"
  Demux5/7 -> Bus Creator5/7  "Vhcl DL2BdyEng x"
  Demux5/6 -> Bus Creator5/6  "Vhcl TrqDL2Bdy1B z"
  Demux5/5 -> Bus Creator5/5  "Vhcl TrqDL2Bdy1B y"
  Demux5/4 -> Bus Creator5/4  "Vhcl TrqDL2Bdy1B x"
  Demux5/3 -> Bus Creator5/3  "Vhcl Trq_DL2Bdy1 z"
  In1/1 -> Demux5/1
  Bus Creator5/1 -> Out1/1
  Demux5/2 -> Bus Creator5/2  "Vhcl Trq_DL2Bdy1 y"
  Demux5/1 -> Bus Creator5/1  "Vhcl Trq_DL2Bdy1 x"

== system AFG_s1v1/TruckMaker/VehicleControl/CreateBus Vhcl.Wheel.In ==
  In1 : Inport
  Bus Creator1 : BusCreator  Inputs=24
  Demux1 : Demux  Outputs=24
      settings: DisplayOption=none
  Out1 : Outport
  wires:
  Demux1/12 -> Bus Creator1/12  "Vhcl Wheel RR rotv"
  Demux1/11 -> Bus Creator1/11  "Vhcl Wheel RR Trq_DL2WC"
  Demux1/10 -> Bus Creator1/10  "Vhcl Wheel RR Trq_B2WC"
  Demux1/9 -> Bus Creator1/9  "Vhcl Wheel RL rotv"
  Demux1/8 -> Bus Creator1/8  "Vhcl Wheel RL Trq_DL2WC"
  Demux1/7 -> Bus Creator1/7  "Vhcl Wheel RL Trq_B2WC"
  Demux1/6 -> Bus Creator1/6  "Vhcl Wheel FR rotv"
  Demux1/5 -> Bus Creator1/5  "Vhcl Wheel FR Trq_DL2WC"
  Demux1/4 -> Bus Creator1/4  "Vhcl Wheel FR Trq_B2WC"
  Demux1/3 -> Bus Creator1/3  "Vhcl Wheel FL rotv"
  Demux1/2 -> Bus Creator1/2  "Vhcl Wheel FL Trq_DL2WC"
  Demux1/1 -> Bus Creator1/1  "Vhcl Wheel FL Trq_B2WC"
  Bus Creator1/1 -> Out1/1
  In1/1 -> Demux1/1
  Demux1/24 -> Bus Creator1/24  "Vhcl Wheel FR2 rotv"
  Demux1/23 -> Bus Creator1/23  "Vhcl Wheel FR2 Trq_DL2WC"
  Demux1/22 -> Bus Creator1/22  "Vhcl Wheel FR2 Trq_B2WC"
  Demux1/21 -> Bus Creator1/21  "Vhcl Wheel FL2 rotv"
  Demux1/20 -> Bus Creator1/20  "Vhcl Wheel FL2 Trq_DL2WC"
  Demux1/19 -> Bus Creator1/19  "Vhcl Wheel FL2 Trq_B2WC"
  Demux1/18 -> Bus Creator1/18  "Vhcl Wheel RR2 rotv"
  Demux1/17 -> Bus Creator1/17  "Vhcl Wheel RR2 Trq_DL2WC"
  Demux1/16 -> Bus Creator1/16  "Vhcl Wheel RR2 Trq_B2WC"
  Demux1/15 -> Bus Creator1/15  "Vhcl Wheel RL2 rotv"
  Demux1/14 -> Bus Creator1/14  "Vhcl Wheel RL2 Trq_DL2WC"
  Demux1/13 -> Bus Creator1/13  "Vhcl Wheel RL2 Trq_B2WC"

== system AFG_s1v1/TruckMaker/VehicleControl/CreateBus VhclCtrl ==
  In : Inport
  BusCreator : BusCreator  Inputs=29
  Demux : Demux  Outputs=29
      settings: DisplayOption=none
  Out : Outport
  wires:
  Demux/29 -> BusCreator/29  "VhclCtrl Lights Reverse"
  Demux/28 -> BusCreator/28  "VhclCtrl Lights Brake"
  Demux/27 -> BusCreator/27  "VhclCtrl Lights FogRear"
  Demux/26 -> BusCreator/26  "VhclCtrl Lights FogFrontR"
  Demux/25 -> BusCreator/25  "VhclCtrl Lights FogFrontL"
  Demux/24 -> BusCreator/24  "VhclCtrl Lights IndR"
  Demux/23 -> BusCreator/23  "VhclCtrl Lights IndL"
  Demux/22 -> BusCreator/22  "VhclCtrl Lights ParkR"
  Demux/21 -> BusCreator/21  "VhclCtrl Lights ParkL"
  Demux/20 -> BusCreator/20  "VhclCtrl Lights Daytime"
  Demux/19 -> BusCreator/19  "VhclCtrl Lights HighBeam"
  Demux/18 -> BusCreator/18  "VhclCtrl Lights LowBeam"
  Demux/17 -> BusCreator/17  "VhclCtrl Steering Trq"
  Demux/16 -> BusCreator/16  "VhclCtrl Steering AngAcc"
  Demux/15 -> BusCreator/15  "VhclCtrl Steering AngVel"
  Demux/14 -> BusCreator/14  "VhclCtrl Steering Ang"
  Demux/13 -> BusCreator/13  "VhclCtrl Gas"
  Demux/12 -> BusCreator/12  "VhclCtrl Clutch"
  Demux/11 -> BusCreator/11  "VhclCtrl BrakePark"
  Demux/10 -> BusCreator/10  "VhclCtrl Brake"
  Demux/9 -> BusCreator/9  "VhclCtrl SelectorCtrl"
  Demux/8 -> BusCreator/8  "VhclCtrl GearNo"
  Demux/7 -> BusCreator/7  "VhclCtrl UserSignal4"
  Demux/6 -> BusCreator/6  "VhclCtrl UserSignal3"
  Demux/5 -> BusCreator/5  "VhclCtrl UserSignal2"
  Demux/4 -> BusCreator/4  "VhclCtrl UserSignal1"
  Demux/3 -> BusCreator/3  "VhclCtrl UserSignal0"
  Demux/2 -> BusCreator/2  "VhclCtrl Key"
  Demux/1 -> BusCreator/1  "VhclCtrl SST"
  BusCreator/1 -> Out/1
  In/1 -> Demux/1

== system AFG_s1v1/TruckMaker/VehicleControl/CreateBus VhclCtrl.PT ==
  In1 : Inport
  BusCreator1 : BusCreator  Inputs=12
  Demux1 : Demux  Outputs=12
      settings: DisplayOption=none
  Out1 : Outport
  wires:
  BusCreator1/1 -> Out1/1
  In1/1 -> Demux1/1
  Demux1/1 -> BusCreator1/1  "VhclCtrl SST"
  Demux1/2 -> BusCreator1/2  "VhclCtrl Key"
  Demux1/3 -> BusCreator1/3  "VhclCtrl UserSignal0"
  Demux1/4 -> BusCreator1/4  "VhclCtrl UserSignal1"
  Demux1/5 -> BusCreator1/5  "VhclCtrl UserSignal2"
  Demux1/6 -> BusCreator1/6  "VhclCtrl UserSignal3"
  Demux1/7 -> BusCreator1/7  "VhclCtrl UserSignal4"
  Demux1/8 -> BusCreator1/8  "VhclCtrl GearNo"
  Demux1/9 -> BusCreator1/9  "VhclCtrl SelectorCtrl"
  Demux1/10 -> BusCreator1/10  "VhclCtrl Clutch"
  Demux1/11 -> BusCreator1/11  "VhclCtrl Gas"
  Demux1/12 -> BusCreator1/12  "VhclCtrl Brake"

== system AFG_s1v1/TruckMaker/VehicleControl/CreateBus VhclCtrl.Steering ==
  In1 : Inport
  Bus Creator : BusCreator  Inputs=5
  Demux : Demux  Outputs=5
      settings: DisplayOption=none
  Out1 : Outport
  wires:
  In1/1 -> Demux/1
  Bus Creator/1 -> Out1/1
  Demux/1 -> Bus Creator/1  "VhclCtrl Steering Ang"
  Demux/5 -> Bus Creator/5  "VhclCtrl Steering ByTrq"
  Demux/3 -> Bus Creator/3  "VhclCtrl Steering AngAcc"
  Demux/2 -> Bus Creator/2  "VhclCtrl Steering AngVel"
  Demux/4 -> Bus Creator/4  "VhclCtrl Steering Trq"

== system AFG_s1v1/TruckMaker/IPG Vehicle/AFGc/1&2 axle ==
  drive torque 1&2 : Inport
  Constant2 : Constant  Value=0
  Gain{,1..3} (4 alike) : Gain  Gain=-1
  To Workspace : ToWorkspace  VariableName=drive_torque1  SampleTime=-1
  Write CM Dict : CarMaker4SL/Write CM Dict  xname=PT.WFL.Trq_Drive  xsync=off
  Write CM Dict1 : CarMaker4SL/Write CM Dict  xname=PT.WFR.Trq_Drive  xsync=off
  Write CM Dict2 : CarMaker4SL/Write CM Dict  xname=PT.WRL.Trq_Drive  xsync=off
  Write CM Dict3 : CarMaker4SL/Write CM Dict  xname=PT.WRR.Trq_Drive  xsync=off
  Write CM Dict4 : CarMaker4SL/Write CM Dict  xname=PT.WFL.Trq_Supp2WC  xsync=off
  Write CM Dict5 : CarMaker4SL/Write CM Dict  xname=PT.WFR.Trq_Supp2WC  xsync=off
  Write CM Dict6 : CarMaker4SL/Write CM Dict  xname=PT.WRL.Trq_Supp2WC  xsync=off
  Write CM Dict7 : CarMaker4SL/Write CM Dict  xname=PT.WRR.Trq_Supp2WC  xsync=off
  Write CM Dict8 : CarMaker4SL/Write CM Dict  xname=PT.Trq_Supp2Bdy1B.y  xsync=off
  Write CM Dict9 : CarMaker4SL/Write CM Dict  xname=PT.Trq_Supp2Bdy1.y  xsync=off
  wires:
  Gain/1 -> Write CM Dict4/1
  Gain1/1 -> Write CM Dict5/1
  Gain2/1 -> Write CM Dict6/1
  Constant2/1 -> Write CM Dict8/1, Write CM Dict9/1
  drive torque 1&2/1 -> Gain/1, Write CM Dict/1, Gain1/1, Write CM Dict1/1, Write CM Dict2/1, Gain2/1, Gain3/1, Write CM Dict3/1, To Workspace/1
  Gain3/1 -> Write CM Dict7/1

== system AFG_s1v1/TruckMaker/IPG Vehicle/AFGc/7&8 axle ==
  drive torque 7&8 : Inport
  Terminator : Terminator  Commented=on
  To Workspace : ToWorkspace  VariableName=drive_torque7_8  SampleTime=-1
  Write CM Dict1 : CarMaker4SL/Write CM Dict  xname=Tr2.Trq_Ext2WhlML  xsync=off
  Write CM Dict2 : CarMaker4SL/Write CM Dict  xname=Tr2.Trq_Ext2WhlRL  xsync=off
  Write CM Dict3 : CarMaker4SL/Write CM Dict  xname=Tr2.Trq_Ext2WhlRR  xsync=off
  Write CM Dict4 : CarMaker4SL/Write CM Dict  xname=Tr2.Trq_Ext2WhlMR  xsync=off
  wires:
  drive torque 7&8/1 -> Write CM Dict1/1, Write CM Dict4/1, Write CM Dict3/1, Write CM Dict2/1, To Workspace/1

== system AFG_s1v1/TruckMaker/IPG Vehicle/AFGc/Subsystem ==
  drive8 : Inport
  Demux1 : Demux  Outputs=8
  Mux : Mux  Inputs=8
  Saturation : Saturate  UpperLimit=3000  LowerLimit=0
  Saturation1 : Saturate  UpperLimit=3000  LowerLimit=0
  Terminator{,1..5} (6 alike) : Terminator
  To Workspace : ToWorkspace  VariableName=drive  SampleTime=-1
  Transfer Fcn1 : TransferFcn  Denominator=[Tst 1]
  Transfer Fcn2 : TransferFcn  Denominator=[Tst 1]
  u1 : Outport
  u3 : Outport  Port=2
  wires:
  Demux1/3 -> Terminator/1, Mux/3
  Demux1/8 -> Saturation1/1
  Demux1/4 -> Terminator1/1, Mux/4
  drive8/1 -> Demux1/1
  Demux1/7 -> Terminator5/1, Mux/7
  Transfer Fcn2/1 -> Mux/8, u3/1
  Demux1/2 -> Mux/2, Terminator4/1
  Demux1/1 -> Saturation/1
  Saturation1/1 -> Transfer Fcn2/1
  Transfer Fcn1/1 -> Mux/1, u1/1
  Saturation/1 -> Transfer Fcn1/1
  Demux1/5 -> Terminator2/1, Mux/5
  Mux/1 -> To Workspace/1
  Demux1/6 -> Terminator3/1, Mux/6

== system AFG_s1v1/TruckMaker/IPG Vehicle/AFGc/brakes ==
  note: torque reverses if wheel goes backwards
  brake torque command : Inport
  wheel speed : Inport  Port=2
  Memory : Memory
  Product : Product
  Rate Limiter : RateLimiter  RisingSlewLimit=brake_rate  FallingSlewLimit=-brake_rate  SampleTimeMode=inherited
  Sign : Signum
  Transport Delay : TransportDelay  Commented=on  DelayTime=brake_lag
  first_order_lags : Subsystem  Commented=on
  Out1 : Outport  VectorParamsAs1DForOutWhenUnconnected=off
  wires:
  Sign/1 -> Product/2
  Product/1 -> Out1/1
  Memory/1 -> Sign/1
  wheel speed/1 -> Memory/1
  Rate Limiter/1 -> Product/1
  Transport Delay/1 -> first_order_lags/1(In1)
  brake torque command/1 -> Rate Limiter/1

== system AFG_s1v1/TruckMaker/IPG Vehicle/AFGc/brakes1 ==
  note: torque reverses if wheel goes backwards
  brake torque command : Inport
  wheel speed : Inport  Port=2
  Memory : Memory
  Product : Product
  Rate Limiter : RateLimiter  RisingSlewLimit=brake_rate  FallingSlewLimit=-brake_rate  SampleTimeMode=inherited
  Sign : Signum
  Transport Delay : TransportDelay  Commented=on  DelayTime=brake_lag
  first_order_lags : Subsystem  Commented=on
  Out1 : Outport  VectorParamsAs1DForOutWhenUnconnected=off
  wires:
  Sign/1 -> Product/2
  Product/1 -> Out1/1
  Memory/1 -> Sign/1
  wheel speed/1 -> Memory/1
  Rate Limiter/1 -> Product/1
  Transport Delay/1 -> first_order_lags/1(In1)
  brake torque command/1 -> Rate Limiter/1
